simulink model "VCUStateflow"  (R2023a)
settings: Solver=FixedStepDiscrete  StartTime=0.0  StopTime=10.0  FixedStep=0.1  RelTol=1e-3  EnableMultiTasking=on
libraries: simulink x1
settings Model: Creator=nickj  LastModifiedBy=nickj
settings SolverCC: AlgebraicLoopSolver=TrustRegion  AutoInsertRateTranBlk=on
settings DataIOCC: LimitDataPoints=on
settings OptimizationCC: LifeSpan=inf
settings DebuggingCC: UnconnectedInputMsg=warning  UnconnectedOutputMsg=warning  UnconnectedLineMsg=warning  AllowSymbolicDim=off  SFUnexpectedBacktrackingDiag=warning  SFNoUnconditionalDefaultTransitionDiag=warning  SFExecutionAtInitializationDiag=none  ArithmeticOperatorsInVariantConditions=warning
settings ModelReferenceCC: EnableRefExpFcnMdlSchedulingChecks=on
settings SFSimCC: SimUseLocalCustomCode=off  CustomCodeUndefinedFunction=UseInterfaceOnly
settings RTWCC: RTWUseLocalCustomCode=off  DLArmComputeVersion=19.05
settings CodeAppCC: StateflowObjectComments=on
settings GRTTargetCC: TargetLangStandard=C89/C90 (ANSI)
settings ConfigComp: CovMetricSettings=dw  CovSaveCumulativeToWorkspaceVar=on  CovSaveSingleToWorkspaceVar=on  CovExternalEMLEnable=off  CovSFcnEnable=off

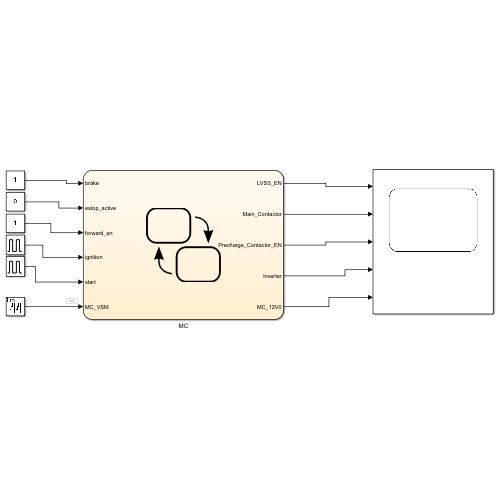
[thumbnail: Simulink's stored preview of the top-level diagram]
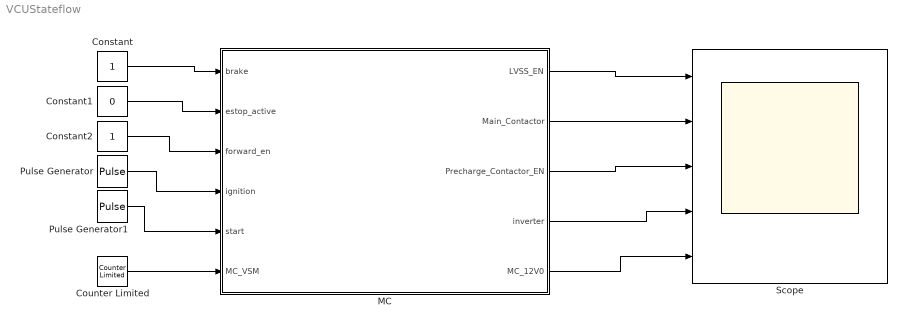
== system VCUStateflow ==
  Constant : Constant
  Constant1 : Constant  Value=0
  Constant2 : Constant
  Counter Limited : simulink/Sources/Counter Limited  uplimit=14  tsamp=3
  MC : Stateflow chart  TreatAsAtomicUnit=on
  Pulse Generator : DiscretePulseGenerator  PulseType=Time based  Period=100  PulseWidth=50
  Pulse Generator1 : DiscretePulseGenerator  PulseType=Time based  Period=50  PulseWidth=50
  Scope : Scope  NumInputPorts=5
  wires:
  Constant/1 -> MC/1(brake)
  Constant1/1 -> MC/2(estop_active)
  Constant2/1 -> MC/3(forward_en)
  Pulse Generator/1 -> MC/4(ignition)
  Pulse Generator1/1 -> MC/5(start)
  Counter Limited/1 -> MC/6(MC_VSM)
  MC/1(LVSS_EN) -> Scope/1
  MC/2(Main_Contactor) -> Scope/2
  MC/3(Precharge_Contactor_EN) -> Scope/3
  MC/4(inverter) -> Scope/4
  MC/5(MC_12V0) -> Scope/5

== stateflow chart VCUStateflow/MC ==
  state ESTOP
    entry:
    MC_12V0 = 0;
    LVSS_EN = 0;
  state MC_Off
    during:
    LVSS_EN = 0;
    MC_12V0 = 0;
  state MC_Discharging
  state Fault
    during:
    LVSS_EN = 1;
    Main_Contactor = 0;
  state MC_Init
    entry:
    LVSS_EN = 1;
    Precharge_Contactor_EN = 1;
  state Contactor_Open
    entry:
    inverter = 0;
    after(20,sec);
    Main_Contactor = 0;
    Precharge_Contactor_EN = 0;
  state Contactor_Closed
    entry:
    Main_Contactor = 1;
    Precharge_Contactor_EN = 0;
    during:
    inverter = 0;
  state MC_Active
    entry:
    inverter = 1;
  note: check
  (default) -> MC_Off
  ESTOP -> MC_Off : [estop_active == 0]
  Fault -> MC_Off [order 1] : [ignition == 0]
  Contactor_Open -> MC_Off
  MC_Off -> MC_Init : [ignition == 1]
  Fault -> MC_Init [order 2] : [MC_VSM ~= 14]
  MC_Init -> Contactor_Open [order 2] : [ignition == 0]
  MC_Init -> Contactor_Closed [order 1] : [MC_VSM == 4]
  MC_Active -> Contactor_Open [order 1] : [ignition == 0]
  Contactor_Closed -> MC_Active : [start == 1 && forward_en == 1 && brake == 1]
  MC_Active -> Contactor_Closed [order 2] : [forward_en == 0]
  data: brake input; estop_active input; forward_en input; ignition input; start input; MC_VSM input; LVSS_EN output; Main_Contactor output; Precharge_Contactor_EN output; inverter output; MC_12V0 output
